simulink model "bpsk7"  (R2021b)
settings: Solver=VariableStepAuto  StartTime=0.0  StopTime=1000  RelTol=1e-3
undefined symbols (not defined in the file): j
libraries: dsp_blocks x7
settings Model: Creator=aidynardabek  LastModifiedBy=aidynardabek

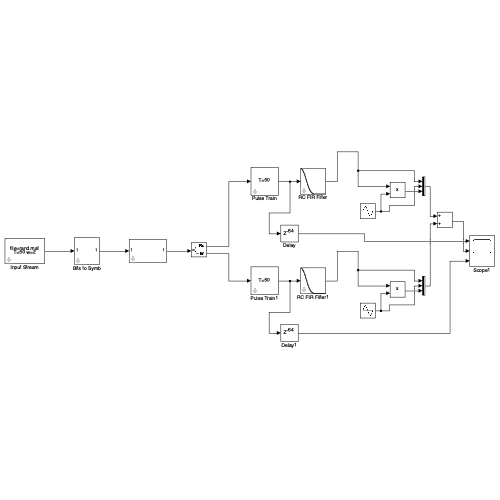
[thumbnail: Simulink's stored preview of the top-level diagram]
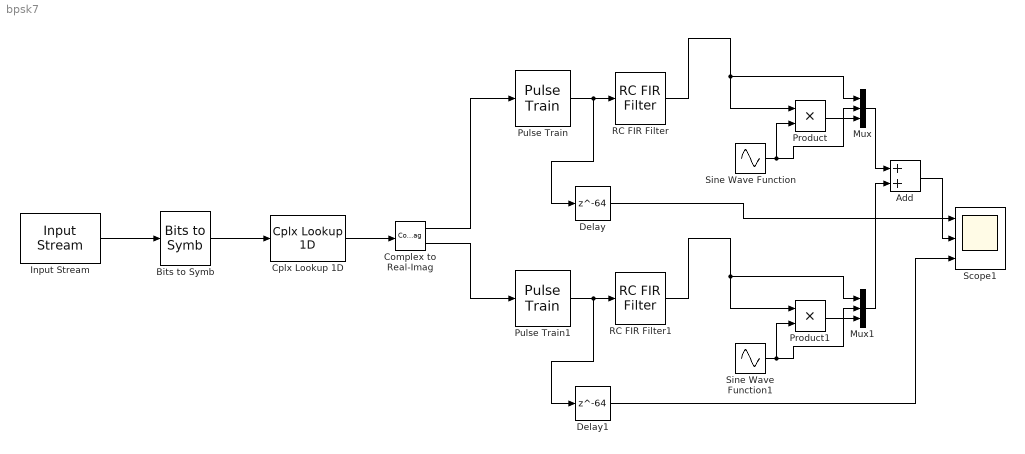
== system bpsk7 ==
  Add : Sum
  Bits to Symb : dsp_blocks/Conversions/Bits to Symb
  Complex to Real-Imag : ComplexToRealImag
  Cplx Lookup 1D : dsp_blocks/Conversions/Cplx Lookup 1D  table=[1 j -1 -j]
  Delay : Delay  DelayLength=64
  Delay1 : Delay  DelayLength=64
  Input Stream : dsp_blocks/Sources//Sinks/Input Stream  period=50  width=2  fname=rand.mat
  Mux : Mux  Inputs=3
  Mux1 : Mux  Inputs=3
  Product : Product
  Product1 : Product
  Pulse Train : dsp_blocks/Conversions/Pulse Train  period=50
  Pulse Train1 : dsp_blocks/Conversions/Pulse Train  period=50
  RC FIR Filter : dsp_blocks/Filters/RC FIR Filter  period=50  beta=0.5  root=off  filt_len=128  win_type=on
  RC FIR Filter1 : dsp_blocks/Filters/RC FIR Filter  period=50  beta=0.5  root=off  filt_len=128  win_type=on
  Scope1 : Scope  NumInputPorts=3
  Sine Wave Function : Sin  Frequency=2*pi*0.1  Phase=pi/2  SampleTime=0
  Sine Wave Function1 : Sin  Frequency=2*pi*0.1  SampleTime=0
  wires:
  Bits to Symb/1 -> Cplx Lookup 1D/1
  Input Stream/1 -> Bits to Symb/1
  Pulse Train/1 -> Delay/1, RC FIR Filter/1
  Delay/1 -> Scope1/1
  Product/1 -> Mux/3
  Sine Wave Function/1 -> Product/2, Mux/2
  RC FIR Filter/1 -> Product/1, Mux/1
  Cplx Lookup 1D/1 -> Complex to Real-Imag/1
  Product1/1 -> Mux1/3
  Sine Wave Function1/1 -> Product1/2, Mux1/2
  Pulse Train1/1 -> Delay1/1, RC FIR Filter1/1
  RC FIR Filter1/1 -> Product1/1, Mux1/1
  Delay1/1 -> Scope1/3
  Complex to Real-Imag/1 -> Pulse Train/1
  Complex to Real-Imag/2 -> Pulse Train1/1
  Mux/1 -> Add/1
  Mux1/1 -> Add/2
  Add/1 -> Scope1/2
